simulink model "rtwdemo_complex"  (Simulink 7.6)
settings: Solver=FixedStepDiscrete  StartTime=0.0  StopTime=10.0  FixedStep=1  RelTol=1e-3
undefined symbols (not defined in the file or in its folder): i
libraries: rtwdemowidgets x1
Description:
  | Efficient Code for Complex Signals
settings Model: Creator=The MathWorks Inc.  ExtModeAutoUpdateStatusClock=off
settings MATStruct: SampleTime=1  Offset=0  Priority=[20.0]
settings DataIOCC: SaveOutput=off  SaveTime=off
settings OptimizationCC: InlineParams=on  InlineInvariantSignals=on  StateBitsets=on  DataBitsets=on  UseTempVars=on  EfficientFloat2IntCast=on  EfficientMapNaN2IntZero=off  BufferReusableBoundary=off
settings DebuggingCC: SolverPrmCheckMsg=none  BusObjectLabelMismatch=none  StrictBusMsg=ErrorOnBusTreatedAsVector
settings HardwareCC: ProdIntDivRoundTo=Zero  ProdEndianess=LittleEndian  ProdHWDeviceType=Generic->32-bit Embedded Processor  TargetHWDeviceType=Generic->32-bit Embedded Processor
settings RTWCC: TLCOptions=-aMaxStackVariableSize=40960  GenerateReport=on  RTWVerbose=off  ProcessScript=grt_make_rtw_hook  LaunchReport=on
settings CodeAppCC: ForceParamTrailComments=on
settings GRTTargetCC: TargetFcnLib=ansi_tfl_tmw.mat

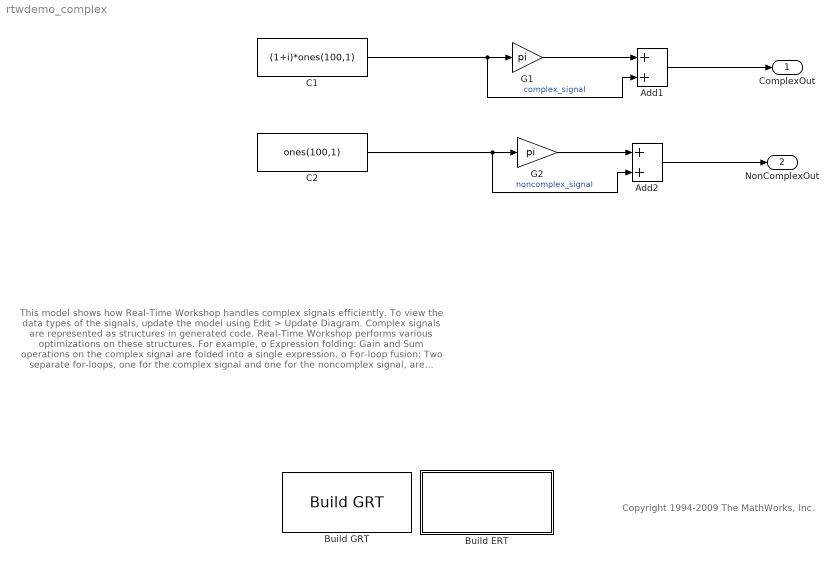
== system rtwdemo_complex ==
  note: This model shows how Real-Time Workshop handles complex signals efficiently.  To
      | view the data types of the signals, update the model using Edit > Update Diagram.
      | Complex signals are represented as structures in generated code. Real-Time Workshop
      | performs various optimizations on these structures.  For example,
      |
      | o Expression folding: Gain and Sum operations on the complex signal are folded into a
      |    single expression.
      | o For-loop fusion: Two separate for-loops, one for the complex signal and one for the
      |    noncomplex signal, are combined into a single for-loop.
      | o Inlined block parameters: The value of Gain block "pi" is inlined in the expression of
      |    the complex Gain-Sum.
      |
      | Because of optimizations such as these, the code generated for complex and noncomplex
      | signals is equally efficient.
  note: Copyright 1994-2009 The MathWorks, Inc.
  Add1 : Sum
  Add2 : Sum
  Build ERT : Subsystem  mask{attrib_overrides={}}
      mask prompts: attrib_overrides "List of attributes to preserve (cell of strings):"
      mask help: Enter the attributes of the configuration set that you want preserved. Otherwise, the default configuration script will override your current settings.
      settings: OpenFcn=|
      | model=bdroot;
      |                   overrides=get_param(gcb,'attrib_overrides');
      | try
      |   rtwconfiguredemo(model,'noop',false,overrides);
      |   set_param(model,'SupportComplex','on');
      |   rtwbuilddemomodel(model);
      | catch
      |   error(lasterr);
      | end; clear model overrides;
      mask Display:
      | disp(['Generate Code Using\n',...
      | 	  'Real-Time Workshop\n',...
      | 	  'Embedded Coder\n'...
      | 	  '(double-click)'])
  Build GRT : rtwdemowidgets/Build GRT  SystemSampleTime=-1  attrib_overrides={}
  C1 : Constant  Value=(1+i)*ones(100,1)  SampleTime=1
  C2 : Constant  Value=ones(100,1)  SampleTime=1
  G1 : Gain  Gain=pi
  G2 : Gain  Gain=pi
  ComplexOut : Outport
  NonComplexOut : Outport  Port=2
  wires:
  C1/1 -> G1/1, Add1/2  "complex_signal"
  G1/1 -> Add1/1
  Add1/1 -> ComplexOut/1
  G2/1 -> Add2/1
  Add2/1 -> NonComplexOut/1
  C2/1 -> G2/1, Add2/2  "noncomplex_signal"

== system rtwdemo_complex/Build ERT ==
